simulink model "motor_simulation"  (R2015a)
settings: Solver=ode45  StartTime=0.0  StopTime=10.0  RelTol=1e-3
undefined symbols (not defined in the file): b, J, Ke, Kt, Ra
libraries: simulink x1
settings Model: Creator=tvincent  LastModifiedBy=tvincent

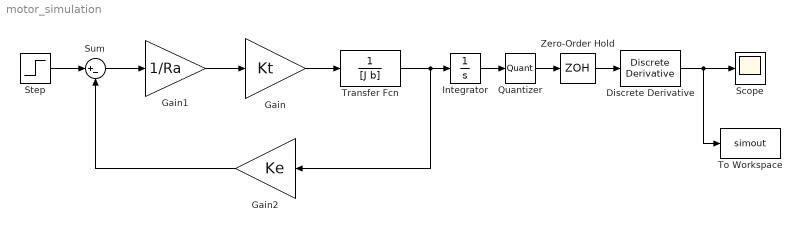
== system motor_simulation ==
  Discrete Derivative : simulink/Discrete/Discrete Derivative  gainval=1.0  ICPrevScaledInput=0.0  InputProcessing=Inherited  OutMin=[]  OutMax=[]  OutDataType=fixdt(1, 16)  OutScaling=2^-10  DoSatur=off
  Gain : Gain  Gain=Kt
  Gain1 : Gain  Gain=1/Ra
  Gain2 : Gain  Gain=Ke
  Integrator : Integrator
  Quantizer : Quantizer  QuantizationInterval=2*pi/3200
  Scope : Scope
  Step : Step  SampleTime=0
  Sum : Sum  Inputs=|+-
  To Workspace : ToWorkspace  VariableName=simout  SaveFormat=Timeseries  SampleTime=-1
  Transfer Fcn : TransferFcn  Denominator=[J b]
  Zero-Order Hold : ZeroOrderHold
  wires:
  Transfer Fcn/1 -> Integrator/1, Gain2/1
  Gain/1 -> Transfer Fcn/1
  Gain1/1 -> Gain/1
  Sum/1 -> Gain1/1
  Gain2/1 -> Sum/2
  Step/1 -> Sum/1
  Integrator/1 -> Quantizer/1
  Discrete Derivative/1 -> To Workspace/1, Scope/1
  Quantizer/1 -> Zero-Order Hold/1
  Zero-Order Hold/1 -> Discrete Derivative/1
